simulink model "fxpdemo_diff"  (Simulink 7.6)
settings: Solver=ode5  SolverMode=SingleTasking  StartTime=0.0  StopTime=10  FixedStep=SampleTime/5  RelTol=1e-3  AbsTol=1e-6
PreLoadFcn:
  | preload_diff
values from neighbouring files (symbols this model uses):
  SampleTime = 0.01    [preload_state_space.m]
undefined symbols (not defined in the file or in its folder): PoleZ
libraries: simulink x4
Description:
  | Fixed-Point Derivatives
  | 
  | Sample implementations of filtered and unfiltered fixed-point derivative algorithms are presented for
  | comparison with floating point implementations.
CloseFcn:
  | close_diff
settings Model: MinMaxOverflowLogging=MinMaxAndOverflow  Creator=The MathWorks Inc.  CovMetricSettings=d  ExtModeTrigMode=oneshot  ExtModeArmWhenConnect=off  ExtModeAutoUpdateStatusClock=off
settings DataIOCC: LimitDataPoints=off  SignalLoggingName=sigsOut
settings OptimizationCC: BooleanDataType=off  InitFltsAndDblsToZero=on  EfficientMapNaN2IntZero=off
settings DebuggingCC: SaveWithParameterizedLinksMsg=none  SignalResolutionControl=TryResolveAllWithWarning  SolverPrmCheckMsg=none  MultiTaskDSMMsg=warning  MultiTaskCondExecSysMsg=none  SigSpecEnsureSampleTimeMsg=none  IntegerOverflowMsg=none  ParameterDowncastMsg=warning  ParameterOverflowMsg=warning  ParameterPrecisionLossMsg=none  StrictBusMsg=None
settings HardwareCC: TargetUnknown=on
settings RTWCC: IncludeERTFirstTime=on
settings GRTTargetCC: TargetFcnLib=ansi_tfl_tmw.mat

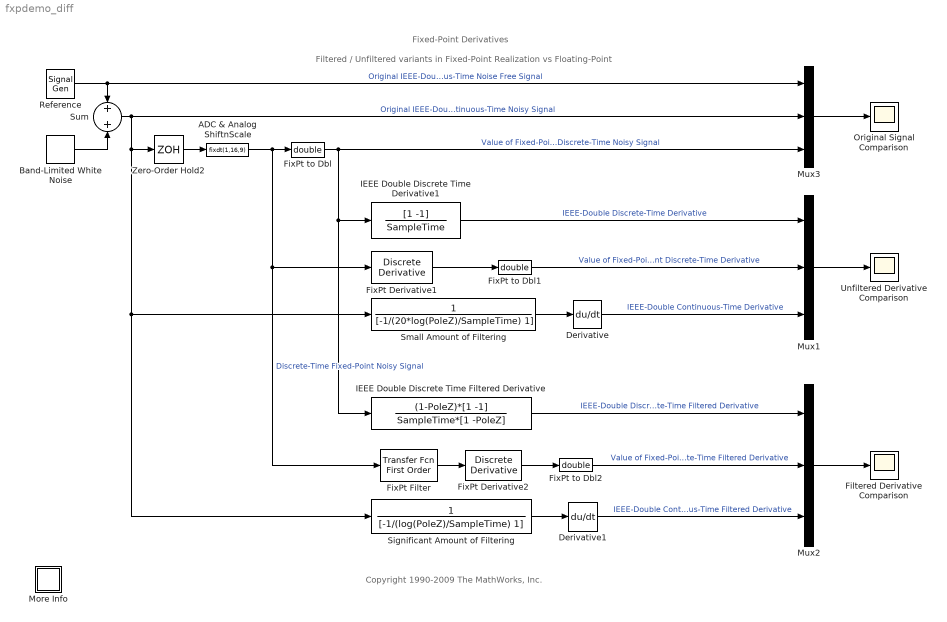
== system fxpdemo_diff ==
  note: Copyright 1990-2009 The MathWorks, Inc.
  note: Filtered / Unfiltered variants in Fixed-Point Realization vs Floating-Point
  note: Fixed-Point Derivatives
  ADC & Analog ShiftnScale : DataTypeConversion  OutDataTypeStr=fixdt(1,16,9)  RndMeth=Nearest  SaturateOnIntegerOverflow=on  LockScale=on
  Band-Limited White Noise : simulink/Sources/Band-Limited White Noise  SystemSampleTime=-1  Cov=[0.0000005]  Ts=SampleTime/5  seed=[23341]
  Derivative : Derivative
  Derivative1 : Derivative
  Filtered Derivative Comparison : Scope
      settings: TickLabels=on  YMin=-3  YMax=3  SaveName=FiltDerivCompare
  FixPt Derivative1 : simulink/Discrete/Discrete Derivative  SystemSampleTime=-1  gainval=1.0  ICPrevScaledInput=0.0  OutMin=[]  OutMax=[]  OutDataType=sfix(16)  OutScaling=2^-10  DoSatur=off
  FixPt Derivative2 : simulink/Discrete/Discrete Derivative  SystemSampleTime=-1  gainval=1.0  ICPrevScaledInput=0.0  OutMin=[]  OutMax=[]  OutDataType=sfix(16)  OutScaling=2^-10  DoSatur=off
  FixPt Filter : simulink/Discrete/Transfer Fcn First Order  SystemSampleTime=-1  PoleZ=PoleZ  ICPrevOutput=0.0  DoSatur=off
  FixPt to Dbl : DataTypeConversion  OutDataTypeStr=double
  FixPt to Dbl1 : DataTypeConversion  OutDataTypeStr=double
  FixPt to Dbl2 : DataTypeConversion  OutDataTypeStr=double
  IEEE Double Discrete Time Derivative1 : DiscreteFilter  Numerator=[1 -1]  Denominator=SampleTime  SampleTime=SampleTime
  IEEE Double Discrete Time Filtered Derivative : DiscreteFilter  Numerator=(1-PoleZ)*[1 -1]  Denominator=SampleTime*[1 -PoleZ]  SampleTime=SampleTime
  More Info : Subsystem
      settings: OpenFcn=showdemo(bdroot(gcs))
      mask Display: disp('?')
  Mux1 : Mux  Inputs=3
  Mux2 : Mux  Inputs=3
  Mux3 : Mux  Inputs=3
  Original Signal Comparison : Scope
      settings: TickLabels=on  YMin=-4  YMax=4  SaveName=OrigSignalCompare
  Reference : SignalGenerator  Amplitude=3  Frequency=0.1*1
  Significant Amount of Filtering : TransferFcn  Denominator=[-1/(log(PoleZ)/SampleTime) 1]
  Small Amount of Filtering : TransferFcn  Denominator=[-1/(20*log(PoleZ)/SampleTime) 1]
  Sum : Sum  Inputs=2  SaturateOnIntegerOverflow=on  InputSameDT=on  OutDataTypeStr=Inherit: Same as first input
  Unfiltered Derivative Comparison : Scope
      settings: TickLabels=on  TimeRange=10  YMin=-3  YMax=3  SaveName=UnfiltDerivCompare
  Zero-Order Hold2 : ZeroOrderHold  SampleTime=SampleTime
  wires:
  Zero-Order Hold2/1 -> ADC & Analog ShiftnScale/1
  ADC & Analog ShiftnScale/1 -> FixPt to Dbl/1, FixPt Filter/1, FixPt Derivative1/1  "Discrete-Time Fixed-Point Noisy Signal"
  FixPt to Dbl/1 -> Mux3/3, IEEE Double Discrete Time Filtered Derivative/1, IEEE Double Discrete Time Derivative1/1  "Value of Fixed-Point Discrete-Time Noisy Signal"
  FixPt Derivative1/1 -> FixPt to Dbl1/1
  FixPt to Dbl1/1 -> Mux1/2  "Value of Fixed-Point Discrete-Time Derivative"
  IEEE Double Discrete Time Derivative1/1 -> Mux1/1  "IEEE-Double Discrete-Time Derivative"
  Derivative/1 -> Mux1/3  "IEEE-Double Continuous-Time Derivative"
  Mux1/1 -> Unfiltered Derivative Comparison/1
  FixPt Filter/1 -> FixPt Derivative2/1
  FixPt to Dbl2/1 -> Mux2/2  "Value of Fixed-Point Discrete-Time Filtered Derivative"
  IEEE Double Discrete Time Filtered Derivative/1 -> Mux2/1  "IEEE-Double Discrete-Time Filtered Derivative"
  Derivative1/1 -> Mux2/3  "IEEE-Double Continuous-Time Filtered Derivative"
  Significant Amount of Filtering/1 -> Derivative1/1
  Mux2/1 -> Filtered Derivative Comparison/1
  Mux3/1 -> Original Signal Comparison/1
  Small Amount of Filtering/1 -> Derivative/1
  Reference/1 -> Sum/1, Mux3/1  "Original IEEE-Double Continuous-Time Noise Free Signal"
  Band-Limited White Noise/1 -> Sum/2
  FixPt Derivative2/1 -> FixPt to Dbl2/1
  Sum/1 -> Mux3/2, Zero-Order Hold2/1, Small Amount of Filtering/1, Significant Amount of Filtering/1  "Original IEEE-Double Continuous-Time Noisy Signal"

== system fxpdemo_diff/More Info ==
